simulink model "Ex4_Mechanical_Model_For_Simulation"  (R2025b)
settings: Solver=VariableStepAuto  StartTime=0.0  StopTime=10.0  RelTol=1e-3
libraries: sm_lib x3, SigiLib x2, nesl_utility x1
settings Model: Creator=resjoehr  LastModifiedBy=resjoehr

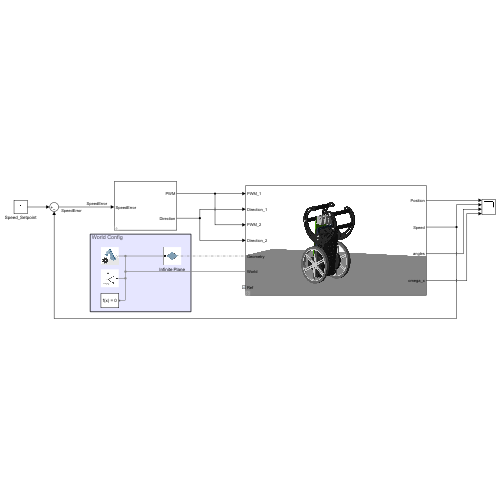
[thumbnail: Simulink's stored preview of the top-level diagram]
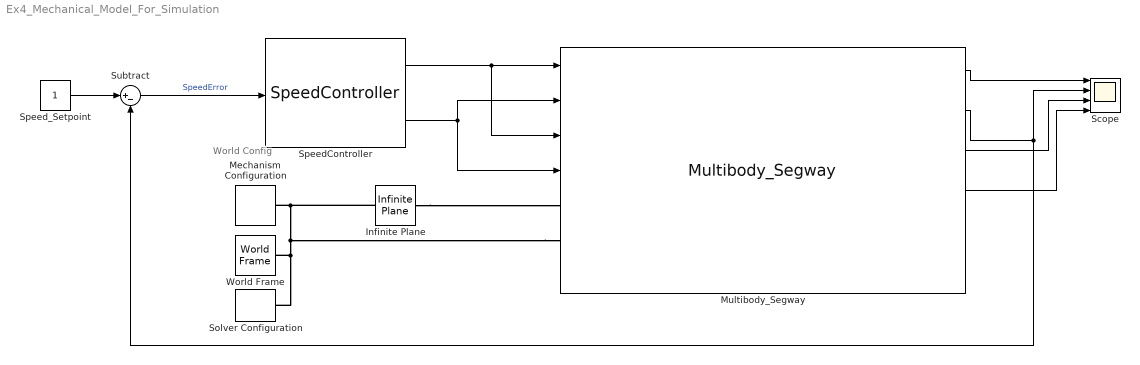
== system Ex4_Mechanical_Model_For_Simulation ==
  note: World Config
  Infinite Plane : sm_lib/Curves and Surfaces/Infinite Plane  GraphicType=Rectangle  GraphicPlaneWidth=1  GraphicPlaneWidthUnits=m  GraphicPlaneHeight=1  GraphicPlaneHeightUnits=m  GraphicVisPropType=SimpleVisualProperties  GraphicDiffuseColor=[0.5 0.5 0.5]  GraphicOpacity=0.25  GraphicSpecularColor=[0.5 0.5 0.5 1.0]  GraphicAmbientColor=[0.15 0.15 0.15 1.0]  GraphicEmissiveColor=[0.0 0.0 0.0 1.0]  GraphicShininess=75
  Mechanism Configuration : sm_lib/Utilities/Mechanism Configuration  UniformGravity=Constant  GravityVector=[0 0 -9.80665]  GravityVectorUnits=m/s^2  LinearizationDelta=0.001  JointModeTransitionNonlinearIterations=2
  Multibody_Segway : SigiLib/Multibody_Segway  Parameter3=motor_left  Parameter2=motor_left
  Scope : Scope  NumInputPorts=4
  Solver Configuration : nesl_utility/Solver Configuration  PhysicalDomain=network_engine_domain  SubClassName=solver  LeftPortType=input  RightPortType=generic  Tones=[]  Harmonics=[]  SimulateNoise=off  Profile=off  UseLocalSampling=off  EnableSwitchedLinearOptims=on  FrequencyDomain=off  UseCCode=off  RelTol=0.001  AbsTol=1e-06  MinStep=1e-09  ToWorkspace=off  RevertToSquareIcSolve=off  NumHomotopyIterations=100  PhasorMode=off  PhasorModeNumHarmonics=1  ConsistencySolver=NEWTON_FTOL  IndexReductionMethod=DerivativeReplacement  DoDC=off  ResidualTolerance=1e-09  ConsistencyTolSource=GLOBAL  ConsistencyAbsTol=0.001  ConsistencyRelTol=0.001  ConsistencyTolFactor=0.001  UseLocalSolver=off  LocalSolverChoice=NE_BACKWARD_EULER_ADVANCER  ResolveIndetEquations=on  FunctionEvalNumThread=1  LocalSolverSampleTime=0.001  DoFixedCost=off  MaxNonlinIter=3  MaxModeIter=2  ComputeImpulses=off  ImpulseIterations=2  LinearAlgebra=Sparse  LinearAlgebraNumThread=0  EquationFormulation=NE_TIME_EF  DelaysMemoryBudget=1024  AutomaticFiltering=on  FilteringTimeConstant=0.001  PartitionStorageMethod=AS_NEEDED  PartitionMemoryBudget=1024  PartitionMethod=FAST  MultibodyUseLocalSolver=off  MultibodyLocalSolverChoice=ODE1  MultibodyLocalSolverSampleTime=0.001
  SpeedController : SigiLib/SpeedController  p_gain=motor_left.P  i_gain=motor_left.I  d_gain=motor_left.D  n_filter=motor_left.N  direction=0
  Speed_Setpoint : Constant
  Subtract : Sum  Inputs=|+-
  World Frame : sm_lib/Frames and Transforms/World Frame
  wires:
  Multibody_Segway/2 -> Scope/2, Subtract/2
  SpeedController/1 -> Multibody_Segway/3, Multibody_Segway/1
  SpeedController/2 -> Multibody_Segway/4, Multibody_Segway/2
  Multibody_Segway/4 -> Scope/4
  Subtract/1 -> SpeedController/1  "SpeedError"
  Speed_Setpoint/1 -> Subtract/1
  Multibody_Segway/1 -> Scope/1
  Multibody_Segway/3 -> Scope/3
  connections:
  Multibody_Segway/LConn2 -- Solver Configuration/RConn1 -- World Frame/RConn1 -- Infinite Plane/LConn1 -- Mechanism Configuration/RConn1
  Infinite Plane/RConn1 -- Multibody_Segway/LConn1
